simulink model "NEW_MAIN"  (R2017b)
settings: Solver=VariableStepAuto  StartTime=0.0  StopTime=10.0  RelTol=1e-3
values from neighbouring files (symbols this model uses):
  A = eye(16,16)    [full_input_list.m]
  B = zeros(16,1)    [full_input_list.m]
  C = blkdiag(eye(3,3),zeros(3,3),eye(10,10))    [full_input_list.m]
  currentMax_B = [0;0.8;0.2]    [full_input_list.m]
  deltaT = 0.00001    (= 1e-05)    [full_input_list.m]
  epsilon_UD_slew = .01    (= 0.01)    [full_input_list.m]
  epsilon_UD_spinUp = .01    (= 0.01)    [full_input_list.m]
  freq = 80    [full_input_list.m]    (also in initSimulink.m)
  H = C    [full_input_list.m]
  I_UD = [0.032808359, 0.000617048, 0.000049185;      0.000617048, 0.032531573, 0.000060042;      0.000049185, 0.000060042, 0.007799591]    [full_input_list.m]
  kd = 0.5    [full_input_list.m]    (also in initACS.m = 0.01)
  kd_UD_detumble = 6e-3    (= 0.006)    [full_input_list.m]
  kp = 1    [full_input_list.m]    (also in initACS.m = 0.01)
  magMomentMax_B = sat2CoilArea.*sat2n.*currentMax_B    [full_input_list.m]
  omega_cmd_N = 1e-1*[1 1 -.6]'    [full_input_list.m]
  omega_spinUp_MAG = 0.05    [full_input_list.m]
  OpModes = [0 0 0]    [full_input_list.m]
  OpTimes = [0 1 2]    [full_input_list.m]
  q4_cmd_init = [q4_cmd_init(2:4); q4_cmd_init(1)]    [full_input_list.m]
  Q_k = zeros(16,16)    [full_input_list.m]
  R = R_k    [full_input_list.m]
  sat2CoilArea = 0.8*[0.02; 0.02; 0.01]    [full_input_list.m]
  sat2n = [0; 100; 100]    [full_input_list.m]
  sat2Resistance = sat2WireLength.*sat2WireResistivity./sat2WireArea    [full_input_list.m]
  SeperationTime = 30000    [full_input_list.m]
  spinAxis_B = [1 0 0]    [full_input_list.m]
  u_k = zeros(16,1)    [full_input_list.m]
  w_k = zeros(16,1)    [full_input_list.m]
  Z_k = zeros(16,1)    [full_input_list.m]
undefined symbols (not defined in the file or in its folder): B_n, B_N, DiscIntNeverNeededParam, G_igrf, gyro_DCM_BS, H_igrf, I_B, IAU, Kschmidt, mag_variance, Orbit_time, R_mean, r_n, r_N, v_n, v_N
libraries: aerolibutil x48, vrlib x37, simulink x22, SimMainLibrary x20, dspmathops x6, sharedtransform x4, dspinverses x2, dspmtrx3 x1, aerolibtransform2 x1, aerolibgravity2 x1, lib_violet_env x1
(part 3 of 3)

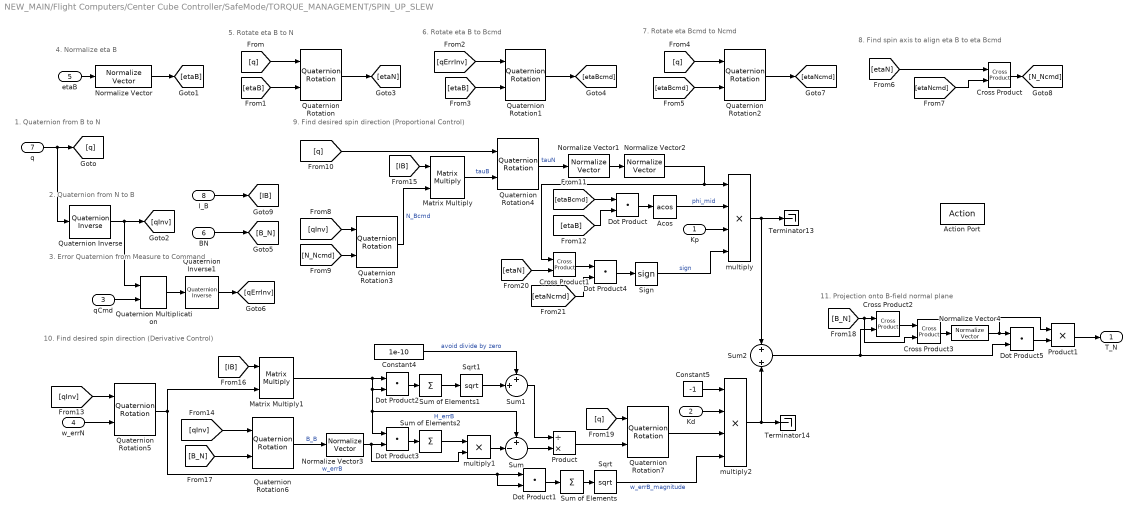
== system NEW_MAIN/Flight Computers/Center Cube Controller/SafeMode/TORQUE_MANAGEMENT/SPIN_UP_SLEW ==
  note: 4. Normalize eta B
  note: 5. Rotate eta B to N
  note: 2. Quaternion from N to B
  note: 7. Rotate eta Bcmd to Ncmd
  note: 8. Find spin axis to align eta B to eta Bcmd
  note: 6. Rotate eta B to Bcmd
  note: 1. Quaternion from B to N
  note: 3. Error Quaternion from Measure to Command
  note: 9. Find desired spin direction (Proportional Control)
  note: 11. Projection onto B-field normal plane
  note: 10. Find desired spin direction (Derivative Control)
  Kp : Inport
  Kd : Inport  Port=2
  qCmd : Inport  Port=3
  w_errN : Inport  Port=4
  etaB : Inport  Port=5
  BN : Inport  Port=6
  q : Inport  Port=7
  I_B : Inport  Port=8
  Action Port : ActionPort  ActionType=case
  Acos : Trigonometry  Operator=acos
  Constant4 : Constant  Value=1e-10
  Constant5 : Constant  Value=-1
  Cross Product{,1..3} (4 alike) : vrlib/Utilities/Cross Product
      settings: SourceProductBaseCode=VR
  Dot Product{,1..5} (6 alike) : DotProduct  InputSameDT=on  OutDataTypeStr=Inherit: Inherit via internal rule
  Matrix Multiply : Product  Multiplication=Matrix(*)
  Matrix Multiply1 : Product  Multiplication=Matrix(*)
  Normalize Vector{,1..4} (5 alike) : vrlib/Utilities/Normalize Vector  maxzero=0
      settings: SourceProductName=Simulink 3D Animation  SourceProductBaseCode=VR
  Product : Product  Inputs=/*
  Product1 : Product
  Quaternion Inverse : aerolibutil/Quaternion Inverse
      settings: SourceProductName=Aerospace Blockset
  Quaternion Inverse1 : aerolibutil/Quaternion Inverse
      settings: SourceProductName=Aerospace Blockset
  Quaternion Multiplication : aerolibutil/Quaternion Multiplication
  Quaternion Rotation{,1..7} (8 alike) : aerolibutil/Quaternion Rotation
  Sign : Signum
  Sqrt : Sqrt  SaturateOnIntegerOverflow=on
  Sqrt1 : Sqrt  SaturateOnIntegerOverflow=on
  Sum : Sum  Inputs=+-|
  Sum of Elements : Sum  Inputs=+
  Sum of Elements1 : Sum  Inputs=+
  Sum of Elements2 : Sum  Inputs=+
  Sum1 : Sum  Inputs=++|
  Sum2 : Sum
  Terminator13 : Terminator
  Terminator14 : Terminator
  multiply : Product  Inputs=****
  multiply1 : Product  Inputs=**
  multiply2 : Product  Inputs=****
  T_N : Outport
  wires:
  [q] -> Quaternion Rotation2/1
  Quaternion Rotation2/1 -> [etaNcmd]
  Normalize Vector3/1 -> Dot Product3/2, multiply1/2
  [qErrInv] -> Quaternion Rotation1/1
  [etaNcmd] -> Cross Product/2
  qCmd/1 -> Quaternion Multiplication/2
  q/1 -> [q], Quaternion Inverse/1
  Sign/1 -> multiply/4  "sign"
  Normalize Vector2/1 -> Cross Product1/1, multiply/1
  [q] -> Quaternion Rotation7/1
  Matrix Multiply1/1 -> Sum/1, Dot Product3/1, Dot Product2/2, Dot Product2/1  "H_errB"
  Dot Product/1 -> Acos/1
  Cross Product3/1 -> Normalize Vector4/1
  Cross Product2/1 -> Cross Product3/1
  Quaternion Rotation7/1 -> multiply2/3
  Sum of Elements/1 -> Sqrt/1
  Quaternion Rotation1/1 -> [etaBcmd]
  [q] -> Quaternion Rotation/1
  [B_N] -> Cross Product2/1, Cross Product3/2
  Normalize Vector/1 -> [etaB]
  Constant4/1 -> Sum1/1  "avoid divide by zero"
  Sqrt1/1 -> Sum1/2
  Sum of Elements1/1 -> Sqrt1/1
  [etaB] -> Quaternion Rotation/2
  Dot Product5/1 -> Product1/2
  Quaternion Rotation/1 -> [etaN]
  [q] -> Quaternion Rotation4/1
  Sum of Elements2/1 -> multiply1/1
  Matrix Multiply/1 -> Quaternion Rotation4/2  "tauB"
  Acos/1 -> multiply/2  "phi_mid"
  w_errN/1 -> Quaternion Rotation5/2
  [etaN] -> Cross Product/1
  [qInv] -> Quaternion Rotation6/1
  Quaternion Rotation5/1 -> Dot Product1/1, Dot Product1/2, Matrix Multiply1/2  "w_errB"
  Sum2/1 -> Cross Product2/2, Dot Product5/2
  [etaBcmd] -> Quaternion Rotation2/2
  Product1/1 -> T_N/1
  Quaternion Rotation4/1 -> Normalize Vector1/1  "tauN"
  [etaN] -> Cross Product1/2
  [qInv] -> Quaternion Rotation3/1
  Constant5/1 -> multiply2/1
  [etaB] -> Quaternion Rotation1/2
  Sum1/1 -> Product/1
  [etaB] -> Dot Product/2
  [IB] -> Matrix Multiply/1
  Dot Product4/1 -> Sign/1
  Quaternion Inverse1/1 -> [qErrInv]
  Cross Product/1 -> [N_Ncmd]
  multiply/1 -> Terminator13/1, Sum2/1
  [B_N] -> Quaternion Rotation6/2
  Quaternion Multiplication/1 -> Quaternion Inverse1/1
  BN/1 -> [B_N]
  [N_Ncmd] -> Quaternion Rotation3/2
  [qInv] -> Quaternion Rotation5/1
  Kp/1 -> multiply/3
  Dot Product3/1 -> Sum of Elements2/1
  Normalize Vector4/1 -> Product1/1, Dot Product5/1
  Normalize Vector1/1 -> Normalize Vector2/1
  etaB/1 -> Normalize Vector/1
  [IB] -> Matrix Multiply1/1
  Dot Product2/1 -> Sum of Elements1/1
  Quaternion Rotation3/1 -> Matrix Multiply/2  "N_Bcmd"
  [etaNcmd] -> Dot Product4/2
  Sum/1 -> Product/2
  Quaternion Inverse/1 -> Quaternion Multiplication/1, [qInv]
  [etaBcmd] -> Dot Product/1
  I_B/1 -> [IB]
  Cross Product1/1 -> Dot Product4/1
  multiply2/1 -> Terminator14/1, Sum2/2
  Dot Product1/1 -> Sum of Elements/1
  Sqrt/1 -> multiply2/4  "w_errB_magnitude"
  multiply1/1 -> Sum/2
  Quaternion Rotation6/1 -> Normalize Vector3/1  "B_B"
  Kd/1 -> multiply2/2
  Product/1 -> Quaternion Rotation7/2

== system NEW_MAIN/Flight Computers/CenterCube EKF/x_measured/Lookup Tables/GPS time to Jd sfrom J2000 ==
  In1 : Inport
  Jd since GPS0 : Constant  Value=2444244.5
  Jd since J2000 : Constant  Value=2451545
  "Leap Seconds from GSP0 " : Constant  Value=27-9
  Sum : Sum  Inputs=|++
  Sum1 : Sum  Inputs=|++
  Sum2 : Sum  Inputs=|+-
  seconds to days conversion : Gain  Gain=1/86400
  Out1 : Outport
  wires:
  In1/1 -> Sum/1
  "Leap Seconds from GSP0 "/1 -> Sum/2
  Sum/1 -> seconds to days conversion/1
  seconds to days conversion/1 -> Sum1/1
  Jd since GPS0/1 -> Sum1/2
  Sum1/1 -> Sum2/1
  Jd since J2000/1 -> Sum2/2
  Sum2/1 -> Out1/1

== system NEW_MAIN/Flight Computers/CenterCube EKF/x_measured/Lookup Tables/Sun position off of Jd frm J2000 ==
  In1 : Inport
  Gain : Gain  Gain=1.49597871e8
  MATLAB Function : MATLAB Function  TreatAsAtomicUnit=on
  Out1 : Outport
  wires:
  In1/1 -> MATLAB Function/1(J2000_days)
  MATLAB Function/1(S_ECI) -> Gain/1
  Gain/1 -> Out1/1

== system NEW_MAIN/Flight Computers/Center Cube Controller/SafeMode/TORQUE_MANAGEMENT/Determine CMD & Error/Quaternion Integration ==
  w_N : Inport
  Integrator1 : Integrator  InitialCondition=q4_cmd_init
  q_normalize : Subsystem
  qderiv : Subsystem
  q4 : Outport
  wires:
  w_N/1 -> qderiv/1(w)
  q_normalize/1(q_out) -> qderiv/2(q), q4/1
  Integrator1/1 -> q_normalize/1(q_in)
  qderiv/1(qd) -> Integrator1/1

== system NEW_MAIN/Flight Computers/Center Cube Controller/SafeMode/TORQUE_MANAGEMENT/Determine CMD & Error/Quaternion Integration/q_normalize ==
  q_in : Inport  PortDimensions=4
  Dot Product : DotProduct  InputSameDT=on  OutDataTypeStr=Inherit: Inherit via internal rule
  Math Function : Math  Operator=sqrt  SaturateOnIntegerOverflow=on
  Product : Product  Inputs=*/  SaturateOnIntegerOverflow=on  InputSameDT=on  OutDataTypeStr=Inherit: Same as first input
  q_out : Outport
  wires:
  Product/1 -> q_out/1
  Math Function/1 -> Product/2
  Dot Product/1 -> Math Function/1
  q_in/1 -> Dot Product/2, Dot Product/1, Product/1

== system NEW_MAIN/Flight Computers/Center Cube Controller/SafeMode/TORQUE_MANAGEMENT/Determine CMD & Error/Quaternion Integration/qderiv ==
  w : Inport
  q : Inport  Port=2
  Mux : Mux  Inputs=2
  Mux1 : Mux
  qd1 : Fcn  Expr=(u(7)*u(1)-u(6)*u(2)+u(5)*u(3))/2
  qd2 : Fcn  Expr=(u(6)*u(1)+u(7)*u(2)-u(4)*u(3))/2
  qd3 : Fcn  Expr=(-u(5)*u(1)+u(4)*u(2)+u(7)*u(3))/2
  qd4 : Fcn  Expr=(-u(4)*u(1)-u(5)*u(2)-u(6)*u(3))/2
  qd : Outport
  wires:
  Mux1/1 -> qd/1
  qd4/1 -> Mux1/4
  qd3/1 -> Mux1/3
  qd2/1 -> Mux1/2
  qd1/1 -> Mux1/1
  Mux/1 -> qd4/1, qd3/1, qd2/1, qd1/1
  q/1 -> Mux/2
  w/1 -> Mux/1

== matlab function NEW_MAIN/Flight Computers/CenterCube EKF/New State Prediction /A_LKF/MATLAB Function ==
  data: A input; A output; replacement input
function A = fcn(A,replacement)
%#codegen
A(13:16,10:12) = replacement;
end

== stateflow chart NEW_MAIN/Flight Computers/PowerBoard Simulation/Chart ==
  state OperationModeDetermination [parallel]
    en, du: ind = max( sum(t>OpTime), 1);
    OM = OpMode( ind );
    settings: executionOrder=2
  note: There should be additional logic added to allow potential ground command override of power board commands (that is, another chart should be added to resolve this issue).
  state SeparationCommand [parallel]
    settings: executionOrder=1
    state NO
      en: SEPC = 0;
    state YES
      en: SEPC = 1;
    NO -> YES : [t > SepTime]
    (default) -> NO
    YES -> NO : [t <= SepTime]
  state GROUND_COMMANDS [parallel]
    en, du: GrdOM = OM;
    GrdSEPC = SEPC;
    settings: executionOrder=3
  data: GrdOM output; GrdSEPC output; t input double; SepTime input double; OpMode input; OpTime input; OM output; SEPC output double; ind local double

== stateflow chart NEW_MAIN/INPUTS/Chart ==
  state INTERPOLATE_STATE
    en,du: r = zeros(3,1);
    v = zeros(3,1);
    B = zeros(3,1);
    ind = 1;
    weight = 1;
    ind = sum(double(t>=T));
    r = r_N(:,ind+1)*weight + r_N(:,ind)*(1-weight);
    v = v_N(:,ind+1)*weight + v_N(:,ind)*(1-weight);
    B = B_N(:,ind+1)*weight + B_N(:,ind)*(1-weight);
  state X = interpTime(T,x,T_curr) [function] [commented out]
  (default) -> INTERPOLATE_STATE
  data: T function_input double size=1; x function_input double size=1; T_curr function_input double size=1; X function_output double size=1; t input; T input; r_N input; v_N input; B_N input; r output; v output; B output; ind local; weight local

== stateflow chart NEW_MAIN/Flight Computers/Center Cube Controller/SafeMode/STATUS_MODE_DETERMINATION ==
  state ADCS_STATUS [parallel]
    en: ErrPos = zeros(1,7);
    settings: executionOrder=1
    state MAGNETOMETER_HEALTH [parallel]
      settings: executionOrder=1
      state BAD
        en: MAG = 0;
        ErrPos(1)=1;
      state OKAY
        en: MAG = 1;
        ErrPos(1)=0;
      ADCS_STATUS.MAGNETOMETER_HEALTH.OKAY -> ADCS_STATUS.MAGNETOMETER_HEALTH.BAD : [Ak(1)==0 && Ak(2) ==0]
      (default) -> ADCS_STATUS.MAGNETOMETER_HEALTH.OKAY
      ADCS_STATUS.MAGNETOMETER_HEALTH.BAD -> ADCS_STATUS.MAGNETOMETER_HEALTH.OKAY : [Ak(1)==1 || Ak(2) ==1]
    state X_TORQUE_STATUS [parallel]
      settings: executionOrder=2
      state BAD
        en: TX = 0;
        ErrPos(5)=1;
      state OKAY
        en: TX = 1;
        ErrPos(5)=0;
      ADCS_STATUS.X_TORQUE_STATUS.OKAY -> ADCS_STATUS.X_TORQUE_STATUS.BAD : [Ak(9) == 0]
      (default) -> ADCS_STATUS.X_TORQUE_STATUS.OKAY
      ADCS_STATUS.X_TORQUE_STATUS.BAD -> ADCS_STATUS.X_TORQUE_STATUS.OKAY : [Ak(9) ==1]
    state ACCELEROMETER_HEALTH [parallel]
      settings: executionOrder=3
      state BAD
        en: ACC = 0;
        ErrPos(2)=1;
      state OKAY
        en: ACC = 1;
        ErrPos(2)=0;
      ADCS_STATUS.ACCELEROMETER_HEALTH.OKAY -> ADCS_STATUS.ACCELEROMETER_HEALTH.BAD : [Ak(3)==0 && Ak(4) ==0]
      (default) -> ADCS_STATUS.ACCELEROMETER_HEALTH.OKAY
      ADCS_STATUS.ACCELEROMETER_HEALTH.BAD -> ADCS_STATUS.ACCELEROMETER_HEALTH.OKAY : [Ak(3)==1 || Ak(4) ==1]
    state Y_TORQUE_STATUS [parallel]
      settings: executionOrder=4
      state BAD
        en: TY = 0;
        ErrPos(6)=1;
      state OKAY
        en: TY = 1;
        ErrPos(6)=0;
      ADCS_STATUS.Y_TORQUE_STATUS.OKAY -> ADCS_STATUS.Y_TORQUE_STATUS.BAD : [Ak(10) == 0]
      (default) -> ADCS_STATUS.Y_TORQUE_STATUS.OKAY
      ADCS_STATUS.Y_TORQUE_STATUS.BAD -> ADCS_STATUS.Y_TORQUE_STATUS.OKAY : [Ak(10) ==1]
    state GYRO_HEALTH [parallel]
      settings: executionOrder=5
      state BAD
        en: GYRO = 0;
        ErrPos(3)=1;
      state OKAY
        en: GYRO = 1;
        ErrPos(3)=0;
      ADCS_STATUS.GYRO_HEALTH.OKAY -> ADCS_STATUS.GYRO_HEALTH.BAD : [Ak(5)==0 && Ak(6) ==0]
      (default) -> ADCS_STATUS.GYRO_HEALTH.OKAY
      ADCS_STATUS.GYRO_HEALTH.BAD -> ADCS_STATUS.GYRO_HEALTH.OKAY : [Ak(5)==1 || Ak(6) ==1]
    state Z_TORQUE_STATUS [parallel]
      settings: executionOrder=6
      state BAD
        en: TZ = 0;
        ErrPos(7)=1;
      state OKAY
        en: TZ = 1;
        ErrPos(7)=0;
      ADCS_STATUS.Z_TORQUE_STATUS.OKAY -> ADCS_STATUS.Z_TORQUE_STATUS.BAD : [Ak(11) == 0]
      (default) -> ADCS_STATUS.Z_TORQUE_STATUS.OKAY
      ADCS_STATUS.Z_TORQUE_STATUS.BAD -> ADCS_STATUS.Z_TORQUE_STATUS.OKAY : [Ak(11) ==1]
    state SUN_SENSOR_HEALTH [parallel]
      settings: executionOrder=7
      state BAD
        en: SS = 0;
        ErrPos(4)=1;
      state OKAY
        en: SS = 1;
        ErrPos(4)=0;
      ADCS_STATUS.SUN_SENSOR_HEALTH.OKAY -> ADCS_STATUS.SUN_SENSOR_HEALTH.BAD : [Ak(7)==0 && Ak(8) ==0]
      (default) -> ADCS_STATUS.SUN_SENSOR_HEALTH.OKAY
      ADCS_STATUS.SUN_SENSOR_HEALTH.BAD -> ADCS_STATUS.SUN_SENSOR_HEALTH.OKAY : [Ak(7)==1 || Ak(8) ==1]
    state OVERALL_STATUS [parallel]
      en, du: Actuator_Health = TX && TY && TZ;
      IMU_Health = MAG && ACC && GYRO && SS;
      settings: executionOrder=8
  state STATE_MACHINE_MODE_DETERMINATION [parallel]
    settings: executionOrder=2
    state INIT
      en, du: SafedOpMode = 0;
      SafeMode_Out = 0;
      PwbMEX = zeros(1,8);
    state TIME_PASSED
      state CALCULATIONS [parallel]
        settings: executionOrder=1
        state SAFE1
          state Case1
            en, du: SafeMode_Out = 0;
            PwbMEX(1) = 0;
            SafedOpMode = PbOpMode;
          state Case2
            en, du: PwbMEX(1) = 1;
            PwbMEX(2:8) = ErrPos;
            SafedOpMode = 11;
          STATE_MACHINE_MODE_DETERMINATION.TIME_PASSED.CALCULATIONS.SAFE1.Case1 -> STATE_MACHINE_MODE_DETERMINATION.TIME_PASSED.CALCULATIONS.SAFE1.Case2 : [PbOpMode == 11]
          (default) -> STATE_MACHINE_MODE_DETERMINATION.TIME_PASSED.CALCULATIONS.SAFE1.Case1
          STATE_MACHINE_MODE_DETERMINATION.TIME_PASSED.CALCULATIONS.SAFE1.Case2 -> STATE_MACHINE_MODE_DETERMINATION.TIME_PASSED.CALCULATIONS.SAFE1.Case1 : [PbOpMode ~= 11]
        state SAFE2
          state Case1
            en, du: SafeMode_Out = 1;
            PwbMEX(1) = 1;
            SafedOpMode = 11;
          state Case2
            en, du: SafedOpMode = 12;
          state Case3
            en, du: SafedOpMode = PbOpMode;
          (default) -> STATE_MACHINE_MODE_DETERMINATION.TIME_PASSED.CALCULATIONS.SAFE2.Case1
          (junction 80) -> STATE_MACHINE_MODE_DETERMINATION.TIME_PASSED.CALCULATIONS.SAFE2.Case1 [order 1] : [IMU_Health==1 || Actuator_Health==1]
          STATE_MACHINE_MODE_DETERMINATION.TIME_PASSED.CALCULATIONS.SAFE2.Case1 -> (junction 80)
          (junction 80) -> STATE_MACHINE_MODE_DETERMINATION.TIME_PASSED.CALCULATIONS.SAFE2.Case2 [order 2] : [EKFHs~=true]
          (junction 80) -> Case3 [order 3] : [EKFHs==true]
          Case3 -> (junction 80)
          STATE_MACHINE_MODE_DETERMINATION.TIME_PASSED.CALCULATIONS.SAFE2.Case2 -> (junction 80)
        (default) -> SAFE1
        SAFE2 -> SAFE1 : [SafeMode_In == true || PbOpMode == 11]
        SAFE1 -> (junction 77) : [~( SafeMode_In == true || PbOpMode == 11 )]
        (junction 77) -> SAFE1 [order 2]
        (junction 77) -> SAFE2 [order 1] : [(OpMode == 5) ||...
            | (OpMode == 6) || ...
            | (OpMode == 7) || ...
            | (OpMode == 9) || ...
            | (OpMode == 10)]
      state UPDATE_MODE [parallel]
        en, du: if (PbOpMode ~= OpMode && OpMode ~= 12)
        SafedOpMode = PbOpMode;
        end
        settings: executionOrder=2
    INIT -> TIME_PASSED : [t>2700]
    (default) -> INIT
  state ATTITUDE_COMPENSATOR_OLD [parallel]
    settings: executionOrder=3
    state UNDEPLOYED [commented out]
      state SLEWING [commented out]
        en, du: T_N = TorquePD_Slew(q,qCmd,etaB,BN,w_errN,KpS,KdS,I_B)
      state DETUMBLING [commented out]
        en, du: T_N = TorqueD(w_BN_N,I_B,q);
      state SEEK_EKF_CONVERGENCE [commented out]
        en: T_N = zeros(1,3);
      state SPIN_UP [commented out]
        en, du: T_N = TorquePD_SpinUp(q,qCmd,etaB,BN,w_errN,KpSU,KdSU,I_B);
      state NULL_DEFAULT [commented out]
        en: T_N = zeros(1,3);
      (junction 184) -> ATTITUDE_COMPENSATOR_OLD.UNDEPLOYED.DETUMBLING [commented out] : [SafedOpMode==5]
      ATTITUDE_COMPENSATOR_OLD.UNDEPLOYED.DETUMBLING -> (junction 184) [commented out]
      ATTITUDE_COMPENSATOR_OLD.UNDEPLOYED.SLEWING -> (junction 184) [commented out]
      (junction 184) -> ATTITUDE_COMPENSATOR_OLD.UNDEPLOYED.SLEWING [commented out] : [SafedOpMode==6]
      (junction 184) -> ATTITUDE_COMPENSATOR_OLD.UNDEPLOYED.SEEK_EKF_CONVERGENCE [commented out] : [SafedOpMode==12]
      ATTITUDE_COMPENSATOR_OLD.UNDEPLOYED.SEEK_EKF_CONVERGENCE -> (junction 184) [commented out]
      (junction 184) -> ATTITUDE_COMPENSATOR_OLD.UNDEPLOYED.SPIN_UP [commented out] : [SafedOpMode==7]
      ATTITUDE_COMPENSATOR_OLD.UNDEPLOYED.NULL_DEFAULT -> (junction 184) [commented out]
      (junction 184) -> ATTITUDE_COMPENSATOR_OLD.UNDEPLOYED.NULL_DEFAULT [commented out]
      ATTITUDE_COMPENSATOR_OLD.UNDEPLOYED.SPIN_UP -> (junction 184) [commented out]
      (default) -> ATTITUDE_COMPENSATOR_OLD.UNDEPLOYED.NULL_DEFAULT [commented out]
    state T_N = TorquePD_Slew(q,qCmd,etaB,BN,w_errN,KpS,KdS,I_B) [function] [commented out]
    state DEPLOYED [commented out]
      state SPIN_UP_SLEW [commented out]
        en, du: T_N = TorqueDeployed(q,w_BN_N);
      state SEEK_EKF_CONVERGENCE [commented out]
        en: T_N = zeros(1,3);
      state NULL_DEFAULT [commented out]
        en: T_N = zeros(1,3);
      (junction 214) -> ATTITUDE_COMPENSATOR_OLD.DEPLOYED.SPIN_UP_SLEW [commented out] : [SafedOpMode==7]
      ATTITUDE_COMPENSATOR_OLD.DEPLOYED.SPIN_UP_SLEW -> (junction 214) [commented out]
      ATTITUDE_COMPENSATOR_OLD.DEPLOYED.SEEK_EKF_CONVERGENCE -> (junction 214) [commented out]
      (junction 214) -> ATTITUDE_COMPENSATOR_OLD.DEPLOYED.SEEK_EKF_CONVERGENCE [commented out] : [SafedOpMode==12]
      ATTITUDE_COMPENSATOR_OLD.DEPLOYED.NULL_DEFAULT -> (junction 214) [commented out]
      (junction 214) -> ATTITUDE_COMPENSATOR_OLD.DEPLOYED.NULL_DEFAULT [commented out]
      (default) -> ATTITUDE_COMPENSATOR_OLD.DEPLOYED.NULL_DEFAULT [commented out]
    state T_N = TorquePD_SpinUp(q,qCmd,etaB,BN,w_errN,KpSU,KdSU,I_B) [function] [commented out]
    state T_N = TorqueDeployed(q,w_BN_N) [function] [commented out]
    state T_N = TorqueD(w_BN_N,I_B,q) [function] [commented out]
    (default) -> ATTITUDE_COMPENSATOR_OLD.UNDEPLOYED [commented out]
    ATTITUDE_COMPENSATOR_OLD.UNDEPLOYED -> ATTITUDE_COMPENSATOR_OLD.DEPLOYED [commented out] : [SEPC==1]
    ATTITUDE_COMPENSATOR_OLD.DEPLOYED -> ATTITUDE_COMPENSATOR_OLD.UNDEPLOYED [commented out] : [SEPC==0]
  state ATTITUDE_COMPENSATOR_NEW [parallel]
    en: MODE = 0;
    settings: executionOrder=4
    state DEPLOYED
      state SPIN_UP_SLEW
        en, du: MODE = 2;
      state NULL_DEFAULT
        en: MODE = 0;
      state SEEK_EKF_CONVERGENCE
        en: MODE = 0;
      (junction 261) -> ATTITUDE_COMPENSATOR_NEW.DEPLOYED.SPIN_UP_SLEW [order 1] : [SafedOpMode==7]
      ATTITUDE_COMPENSATOR_NEW.DEPLOYED.SPIN_UP_SLEW -> (junction 261)
      (junction 261) -> ATTITUDE_COMPENSATOR_NEW.DEPLOYED.NULL_DEFAULT [order 3]
      ATTITUDE_COMPENSATOR_NEW.DEPLOYED.NULL_DEFAULT -> (junction 261)
      ATTITUDE_COMPENSATOR_NEW.DEPLOYED.SEEK_EKF_CONVERGENCE -> (junction 261)
      (default) -> ATTITUDE_COMPENSATOR_NEW.DEPLOYED.NULL_DEFAULT
      (junction 261) -> ATTITUDE_COMPENSATOR_NEW.DEPLOYED.SEEK_EKF_CONVERGENCE [order 2] : [SafedOpMode==12]
    state UNDEPLOYED
      state SLEWING
        en, du: MODE = 1;
        KP = KpS; KD = KdS;
      state DETUMBLING
        en, du: MODE = 3;
      state NULL_DEFAULT
        en: MODE = 0;
      state SEEK_EKF_CONVERGENCE
        en: MODE = 0;
      state SPIN_UP
        en, du: MODE = 1;
        KP = KpSU; KD = KdSU;
      (junction 233) -> ATTITUDE_COMPENSATOR_NEW.UNDEPLOYED.DETUMBLING [order 1] : [SafedOpMode==5]
      ATTITUDE_COMPENSATOR_NEW.UNDEPLOYED.DETUMBLING -> (junction 233)
      ATTITUDE_COMPENSATOR_NEW.UNDEPLOYED.SLEWING -> (junction 233)
      (junction 233) -> ATTITUDE_COMPENSATOR_NEW.UNDEPLOYED.SLEWING [order 2] : [SafedOpMode==6]
      (junction 233) -> ATTITUDE_COMPENSATOR_NEW.UNDEPLOYED.NULL_DEFAULT [order 5]
      ATTITUDE_COMPENSATOR_NEW.UNDEPLOYED.NULL_DEFAULT -> (junction 233)
      (junction 233) -> ATTITUDE_COMPENSATOR_NEW.UNDEPLOYED.SPIN_UP [order 3] : [SafedOpMode==7]
      ATTITUDE_COMPENSATOR_NEW.UNDEPLOYED.SEEK_EKF_CONVERGENCE -> (junction 233)
      (default) -> ATTITUDE_COMPENSATOR_NEW.UNDEPLOYED.NULL_DEFAULT
      (junction 233) -> ATTITUDE_COMPENSATOR_NEW.UNDEPLOYED.SEEK_EKF_CONVERGENCE [order 4] : [SafedOpMode==12]
      ATTITUDE_COMPENSATOR_NEW.UNDEPLOYED.SPIN_UP -> (junction 233)
    ATTITUDE_COMPENSATOR_NEW.DEPLOYED -> ATTITUDE_COMPENSATOR_NEW.UNDEPLOYED : [SEPC==0]
    (default) -> ATTITUDE_COMPENSATOR_NEW.UNDEPLOYED
    ATTITUDE_COMPENSATOR_NEW.UNDEPLOYED -> ATTITUDE_COMPENSATOR_NEW.DEPLOYED : [SEPC==1]
  data: q function_input double size=1; qCmd function_input double size=1; etaB function_input double size=1; BN function_input double size=1; w_errN function_input double size=1; KpS function_input double size=1; KdS function_input double size=1; I_B function_input double size=1; T_N function_output double size=1; q function_input double size=1; qCmd function_input double size=1; etaB function_input double size=1; BN function_input double size=1; w_errN function_input double size=1; KpSU function_input double size=1; KdSU function_input double size=1; I_B function_input double size=1; T_N function_output double size=1; q function_input double size=1; w_BN_N function_input double size=1; T_N function_output double size=1; w_BN_N function_input double size=1; I_B function_input double size=1; q function_input double size=1; T_N function_output double size=1; MODE output; KP output; KD output; Ak input; PbOpMode input; SEPC input; ErrPos local; MAG output; ACC output; GYRO output; SS output; TX output; TY output; TZ output; Actuator_Health output; IMU_Health output; t input; SafeMode_In input; EKFHs input; SafeMode_Out output; PwbMEX output; SafedOpMode output; KpS input; KpSU input; KdS input; KdSU input; OpMode input; SepCmd input

== matlab function NEW_MAIN/Flight Computers/CenterCube EKF/x_measured/q_N from Sensors/quat From DCM ==
  data: Q input; q_N output; D output
function [q_N,D]  = fcn(Q)

    [V,D] = eig(Q);
    q_N = zeros(4,1);
    a = zeros(3,1);
    tol = 1e-10;
    
    if abs(real(D(1,1))-1) <= tol
        a(:,1) = real(V(:,1));
        phi = atan(abs(imag(D(2,2)))/real(D(2,2)));
    elseif abs(real(D(2,2))-1) <= tol
        a(:,1) = real(V(:,2));
        phi = atan(abs(imag(D(1,1)))/real(D(1,1)));
    elseif abs(real(D(3,3))-1) <= tol
        a(:,1) = real(V(:,3));
        phi = atan(abs(imag(D(1,1)))/real(D(1,1)));
    else 
        a(:,1) = [1;0;0];
        phi = 0;
    end
    
    q_N(1) = a(1)*sin(phi/2);
    q_N(2) = a(2)*sin(phi/2);
    q_N(3) = a(3)*sin(phi/2);
    q_N(4) = cos(phi/2);
end

== matlab function NEW_MAIN/Flight Computers/CenterCube EKF/New State Prediction /Predictions ==
  data: x_ko input; F output; x_kp output
function [F,x_kp] = fcn(x_ko)
%#codegen

% BASIC 
GM = 3.986e14;
%% EOMs:
% xdd = - GM*x/(x^2+y^2+z^2)^(3/2)
% ydd = - GM*y/(x^2+y^2+z^2)^(3/2)
% zdd = - GM*z/(x^2+y^2+z^2)^(3/2)
n = length(x_ko);
x = x_ko(1);
y = x_ko(2);
z = x_ko(3);

w1 = x_ko(n-6);
w2 = x_ko(n-5);
w3 = x_ko(n-4);
q1 = x_ko(n-3);
q2 = x_ko(n-2);
q3 = x_ko(n-1);
q4 = x_ko(n);

x_kp = zeros(n,1);
F = zeros(n,n);

%% predicted state estimate
x_kp(1) = x_ko(4);
x_kp(2) = x_ko(5);
x_kp(3) = x_ko(6);
x_kp(4) = -GM*x/(x^2+y^2+z^2)^(3/2); 
x_kp(5) = -GM*y/(x^2+y^2+z^2)^(3/2);
x_kp(6) = -GM*z/(x^2+y^2+z^2)^(3/2);

x_kp(n-3) = 0.5*(w1*q4-q3*w2+q2*w3);
x_kp(n-2) = 0.5*(w1*q3+q4*w2-q1*w3);
x_kp(n-1) = 0.5*(-w1*q2+q1*w2+q4*w3);
x_kp(n) = 0.5*(-w1*q1-q2*w2-q3*w3);

%% F matrix for predicted covariance estimate 
% F for x
F(1,4) = 1;
F(2,5) = 1;
F(3,6) = 1;
% F for xdot
F(4,4) = (3/2)*(2*x^2)/(x^2+y^2+z^2)^(5/2)-1/(x^2+y^2+z^2)^(3/2);
F(4,5) = (3/2)*2*x*y/(x^2+y^2+z^2)^(5/2);
F(4,6) = (3/2)*2*x*z/(x^2+y^2+z^2)^(5/2);

F(5,4) = (3/2)*2*x*y/(x^2+y^2+z^2)^(5/2);
F(5,5) = (3/2)*(2*y^2)/(x^2+y^2+z^2)^(5/2)-1/(x^2+y^2+z^2)^(3/2);
F(5,6) = (3/2)*2*y*z/(x^2+y^2+z^2)^(5/2);

F(6,4) = (3/2)*2*x*z/(x^2+y^2+z^2)^(5/2);
F(6,5) = (3/2)*2*y*z/(x^2+y^2+z^2)^(5/2);
F(6,6) = (3/2)*(2*z^2)/(x^2+y^2+z^2)^(5/2)-1/(x^2+y^2+z^2)^(3/2);

% F for xddot
% Leave as 0 to ensure no changes in thetadot
% 7-8-9

% F for thetadot
% Leave as 0 to ensure no changes in thetadot
% 10-11-12

% F for quaternion changes
F(n-3,n-6) = 0.5*q4;
F(n-3,n-5) = -0.5*q3;
F(n-3,n-4) = 0.5*q2;
F(n-3,n-3) = 0;
F(n-3,n-2) = 0.5*w3;
F(n-3,n-1) = -0.5*w2;
F(n-3,n) = 0.5*w1;

F(n-2,n-6) = 0.5*q3;
F(n-2,n-5) = 0.5*q4;
F(n-2,n-4) = -0.5*q1;
F(n-2,n-3) = -0.5*w3;
F(n-2,n-2) = 0;
F(n-2,n-1) = 0.5*w1;
F(n-2,n) = 0.5*w2;

F(n-1,n-6) = -0.5*q2;
F(n-1,n-5) = 0.5*q1;
F(n-1,n-4) = 0.5*q4;
F(n-1,n-3) = 0.5*w2;
F(n-1,n-2) = -0.5*w1;
F(n-1,n-1) = 0;
F(n-1,n) = 0.5*w3;

F(n,n-6) = -0.5*q1;
F(n,n-5) = -0.5*q2;
F(n,n-4) = -0.5*q3;
F(n,n-3) = -0.5*w1;
F(n,n-2) = -0.5*w2;
F(n,n-1) = -0.5*w3;
F(n,n) = 0;
end

== matlab function NEW_MAIN/Sensors/Center Cube Sensors/Gyro/Bias ==
  data: w input; wn output; noise input
function wn = fcn(w, noise)
%#codegen
    
    % Add the bias to the rotation rate.
    wn = zeros(size(noise));
    for k = 1:size(noise, 2)
        wn(:, k) = w + noise(:, k);
    end
    
end

== matlab function NEW_MAIN/Sensors/Center Cube Sensors/Create Sun Vector/MATLAB Function ==
  data: J2000_days input; S_ECI output
function S_ECI = sun_position(J2000_days)
% SUN_ECI  Calculate the cartesian coordinates of the sun (in AU)
%			  in the Earth Centered Inertial (ECI) reference frame
%			  with mean equator and equinox of J2000
%
% [S_ECI] = SUN_ECI(J2000_days)
%
% Arguments:
% J2000_days 	- UT Days elapsed since J2000 (1 January, 2000, 12 noon)
% S_ECI				- Sun vector in ECI, units of AU
%
% Todd Humphreys
% Author: Todd Humphreys
% Algorithm: Modified algorithm based on Astronomical Almanac 2001, pg C24
% Tested: Todd Humphreys, November 10, 2001
% 			 Within 0.01 degrees of ECI sun vector from Astronomical Almanac 


RAD = 57.29577951308232;

T   = (J2000_days)/36525;		% Julian centuries since J2000
L0  = (280.46645 + 36000.76983*T + 0.0003032*T^2)/RAD;	% Mean longitude of Sun
M   = (357.52910 + 35999.05030*T - 0.0001559*T^2 - 0.00000048*T^3)/RAD;	 % Mean anomaly
e   = 0.016708617 - 0.000042037*T - 0.0000001236*T^2;
C   = (1.914600 - 0.004817*T - 0.000014*T^2)*sin(M) + (0.019993 - 0.000101*T)*sin(2*M) + 0.000290*sin(3*M);
C   = C/RAD;
SL  = L0 + C;	% Ecliptic longitude
Ni  = M + C;	% Sun true Anomaly
R   = 1.000001018*(1-e^2)/(1+e*cos(Ni));  % Distance, Earth to Sun
SL = SL - (0.01397*T*100)/RAD;	% Correction to ecliptic longitude to reference to J200 equinox
Obl = (23.439291 - 0.0130042*T - 0.00000016*T^2 + 0.000000504*T^3)/RAD;	% Obliquity of ecliptic
SL     = (SL/(2*pi) - floor(SL/(2*pi)))*2*pi;	% Reduce to 2pi range
RA     = atan2(cos(Obl)*sin(SL),cos(SL));		% Right ascension	
Dec    = asin(sin(Obl).*sin(SL));				% Declination

S_ECI = [R*cos(SL); R*cos(Obl)*sin(SL); R*sin(Obl)*sin(SL)];

== matlab function NEW_MAIN/Flight Computers/CenterCube EKF/x_measured/Lookup Tables/Sun position off of Jd frm J2000/MATLAB Function ==
  data: J2000_days input; S_ECI output
function S_ECI = sun_position(J2000_days)
% SUN_ECI  Calculate the cartesian coordinates of the sun (in AU)
%			  in the Earth Centered Inertial (ECI) reference frame
%			  with mean equator and equinox of J2000
%
% [S_ECI] = SUN_ECI(J2000_days)
%
% Arguments:
% J2000_days 	- UT Days elapsed since J2000 (1 January, 2000, 12 noon)
% S_ECI				- Sun vector in ECI, units of AU
%
% Todd Humphreys
% Author: Todd Humphreys
% Algorithm: Modified algorithm based on Astronomical Almanac 2001, pg C24
% Tested: Todd Humphreys, November 10, 2001
% 			 Within 0.01 degrees of ECI sun vector from Astronomical Almanac 


RAD = 57.29577951308232;

T   = (J2000_days)/36525;		% Julian centuries since J2000
L0  = (280.46645 + 36000.76983*T + 0.0003032*T^2)/RAD;	% Mean longitude of Sun
M   = (357.52910 + 35999.05030*T - 0.0001559*T^2 - 0.00000048*T^3)/RAD;	 % Mean anomaly
e   = 0.016708617 - 0.000042037*T - 0.0000001236*T^2;
C   = (1.914600 - 0.004817*T - 0.000014*T^2)*sin(M) + (0.019993 - 0.000101*T)*sin(2*M) + 0.000290*sin(3*M);
C   = C/RAD;
SL  = L0 + C;	% Ecliptic longitude
Ni  = M + C;	% Sun true Anomaly
R   = 1.000001018*(1-e^2)/(1+e*cos(Ni));  % Distance, Earth to Sun
SL = SL - (0.01397*T*100)/RAD;	% Correction to ecliptic longitude to reference to J200 equinox
Obl = (23.439291 - 0.0130042*T - 0.00000016*T^2 + 0.000000504*T^3)/RAD;	% Obliquity of ecliptic
SL     = (SL/(2*pi) - floor(SL/(2*pi)))*2*pi;	% Reduce to 2pi range
RA     = atan2(cos(Obl)*sin(SL),cos(SL));		% Right ascension	
Dec    = asin(sin(Obl).*sin(SL));				% Declination

S_ECI = [R*cos(SL); R*cos(Obl)*sin(SL); R*sin(Obl)*sin(SL)];
